simulink model "func_findClosestTrajectoryIndex"  (R2024a)
settings: configuration reference "SharedConfig" (kept outside this file)
undefined symbols (not defined in the file or in its folder): num_of_wps
settings Model: DataDictionary=configuration_dictionary.sldd  Creator=ander  LastModifiedBy=matlab.cut
settings ConfigSetRef: SourceName=SharedConfig

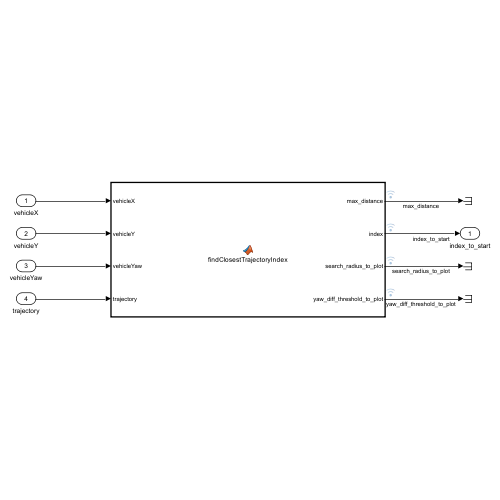
[thumbnail: Simulink's stored preview of the top-level diagram]
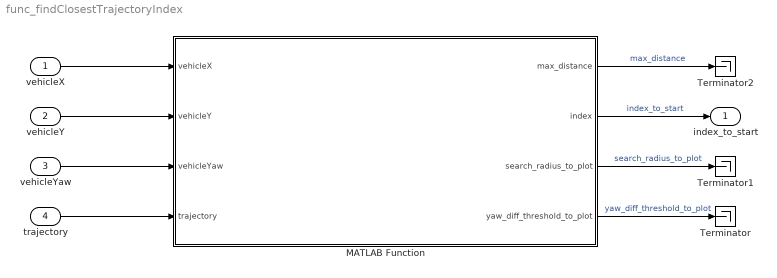
== system func_findClosestTrajectoryIndex ==
  vehicleX : Inport  OutDataTypeStr=double  PortDimensions=[1 1]
  vehicleY : Inport  Port=2  OutDataTypeStr=double  PortDimensions=[1 1]
  vehicleYaw : Inport  Port=3  OutDataTypeStr=double  PortDimensions=[1 1]
  trajectory : Inport  Port=4  OutDataTypeStr=double  PortDimensions=[num_of_wps 3]
  MATLAB Function : MATLAB Function  TreatAsAtomicUnit=on
  Terminator : Terminator
  Terminator1 : Terminator
  Terminator2 : Terminator
  index_to_start : Outport  OutDataTypeStr=double  PortDimensions=1
  wires:
  vehicleX/1 -> MATLAB Function/1(vehicleX)
  vehicleY/1 -> MATLAB Function/2(vehicleY)
  vehicleYaw/1 -> MATLAB Function/3(vehicleYaw)
  trajectory/1 -> MATLAB Function/4(trajectory)
  MATLAB Function/1(max_distance) -> Terminator2/1  "max_distance"
  MATLAB Function/2(index) -> index_to_start/1  "index_to_start"
  MATLAB Function/3(search_radius_to_plot) -> Terminator1/1  "search_radius_to_plot"
  MATLAB Function/4(yaw_diff_threshold_to_plot) -> Terminator/1  "yaw_diff_threshold_to_plot"

== matlab function func_findClosestTrajectoryIndex/MATLAB Function ==
  data: vehicleX input; vehicleY input; vehicleYaw input; trajectory input; max_distance output; index output; search_radius_to_plot output; L parameter; yaw_diff_threshold_to_plot output
function [max_distance, index, search_radius_to_plot, yaw_diff_threshold_to_plot] = findClosestTrajectoryIndex(vehicleX, vehicleY, vehicleYaw, trajectory, L)
    % Initialize variables
    max_distance = -inf;
    index = 0;
    search_radius = L;
    search_radius_to_plot = 0;
    yaw_diff_threshold_to_plot = 0; 


    while index == 0 && search_radius <= 10*L
       
       if search_radius <= 2*L
           yaw_diff_threshold = 40;
       elseif search_radius <= 5*L
           yaw_diff_threshold = 30;       
       else
           yaw_diff_threshold = 20;
       end


       for i = 1:size(trajectory, 1)-1
          % Coordinates and yaw of the line segment endpoints
          point1X = trajectory(i, 1);
          point1Y = trajectory(i, 2);
          point2X = trajectory(i+1, 1);
          point2Y = trajectory(i+1, 2);

          % Find the intersection between the line segment and a circle around the vehicle
          [x_inter, y_inter, line_segment_angle] = intersectLineCircle(point1X, point1Y, point2X, point2Y, vehicleX, vehicleY, search_radius);

          % Check if the intersection point is ahead of the vehicle
          if ~isempty(x_inter) && ~isempty(y_inter)
              vec_to_intersection = [x_inter - vehicleX, y_inter - vehicleY];
              vehicle_dir = [cosd(vehicleYaw), sind(vehicleYaw)];
              dot_product = dot(vec_to_intersection, vehicle_dir);
              
              % line segment angle
              if line_segment_angle < 0
                  line_segment_angle = line_segment_angle + 360;
              end

              % Calcula a diferença de YAW entre o veículo e o ponto atual
              vehicleYaw_to_trajectorySegmentYaw  = abs(vehicleYaw - line_segment_angle);

              % angle between the vector from the vehicle's position to the intersection point 
              intersection_angle_deg = atan2d(y_inter - vehicleY, x_inter - vehicleX);

              if intersection_angle_deg(1) < 0
                  intersection_angle_deg(1) = intersection_angle_deg(1) + 360;
              end
              
               % disp('check')
               % disp(i)
               % disp(search_radius)
               % disp(yaw_diff_threshold)
               % disp(dot_product)
               % disp(vehicleYaw)
               % disp(line_segment_angle)
               % disp(abs(vehicleYaw - intersection_angle_deg(1)))
               % disp(abs(vehicleYaw_to_trajectorySegmentYaw))

              % Check if the intersection is ahead of the vehicle and within the yaw threshold
              if dot_product(1) > 0 && ...
                      abs(vehicleYaw - intersection_angle_deg(1)) <= yaw_diff_threshold && ...
                      abs(vehicleYaw_to_trajectorySegmentYaw) <= yaw_diff_threshold 

                  distance_to_point = norm(vec_to_intersection);
                  
                  % disp('index')              
                  % disp(i)
                  % disp( vehicleYaw )
                  % disp(line_segment_angle)    
                  % disp(vec_to_intersection)
                  % disp(vehicle_dir)
                  % disp(dot_product(1) )
                  % disp('') 
                  
                  % Update the max distance and index if this point is farther away
                  if distance_to_point > max_distance
                      max_distance = distance_to_point;
                      index = i;
                      search_radius_to_plot = search_radius;
                      yaw_diff_threshold_to_plot = yaw_diff_threshold;
                  end
              end
          end
       end

       % Increase the search radius if no valid point is found
       if index == 0
           search_radius = search_radius + 0.5;
       end
    end
end




%% intersectLineCircle
function [x_inter, y_inter, line_segment_angle] = intersectLineCircle(x1, y1, x2, y2, h, k, r)
    a = (y2-y1) / (x2-x1);
    b = y1 - a*x1;
    line_segment_angle = atan2d(y2-y1,x2-x1);

    
    x_inter = [0,0];
    y_inter = [0,0];

    % Encontrar os pontos de interseção
    A = 1 + a^2;
    B = 2*(a*b - a*k - h);
    C = h^2 + b^2 + k^2 -2*b*k - r^2;

    delta = B^2 - 4*A*C;

    if delta < 0
        x_inter = [];
        y_inter = [];
        return;
    end

    x_inter(1) = (-B + sqrt(delta)) / (2*A);
    x_inter(2) = (-B - sqrt(delta)) / (2*A);

    y_inter(1) = a*x_inter(1) + b;
    y_inter(2) = a*x_inter(2) + b;
    
        
    % Verificar se os pontos de interseção estão dentro do segmento de reta
    if ((x_inter(1)-x1)*(x_inter(1)-x2) <= 0) && ((y_inter(1)-y1)*(y_inter(1)-y2) <= 0)
        % disp('pontos de interseção - ahead');
        x_inter = x_inter(1);
        y_inter = y_inter(1);
        
    elseif ((x_inter(2)-x1)*(x_inter(2)-x2) <= 0) && ((y_inter(2)-y1)*(y_inter(2)-y2) <= 0)
        % disp('pontos de interseção - behind');
        x_inter = x_inter(2);
        y_inter = y_inter(2);

    else
        x_inter = [];
        y_inter = [];
    end
end
